simulink model "MIEM_Adaptive"  (Simulink 7.8)
settings: Solver=ode1  StartTime=0.0  StopTime=inf  FixedStep=0.001  RelTol=1e-3
undefined symbols (not defined in the file): HIL, qc_get_step_size
libraries: quarc_library x39, simulink x20, dspmtrx3 x3
(part 1 of 2)
settings Model: Creator=danso  LastModifiedBy=danso  SimulationMode=external  ExtModeTrigDuration=5000
settings SolverCC: PositivePriorityOrder=on
settings RTWCC: SystemTargetFile=quarc_win64.tlc  TemplateMakefile=quarc_default_tmf  Description=QUARC Win64 Target  ProcessScript=quarc_win64_make_rtw_hook
settings STFCustomTargetCC: TargetPreCompLibLocation=C:\PROGRA~3\QUARC\lib\2011b\win64\release  SystemTargetFile=quarc_win64.tlc
settings GRTTargetCC: TargetPreCompLibLocation=C:\PROGRA~3\QUARC\lib\2011b\win64\release  ParMdlRefBuildCompliant=off  CompOptLevelCompliant=off  ConcurrentExecutionCompliant=off  MatFileLogging=off  ExtMode=on  ExtModeMexFile=quarc_comm

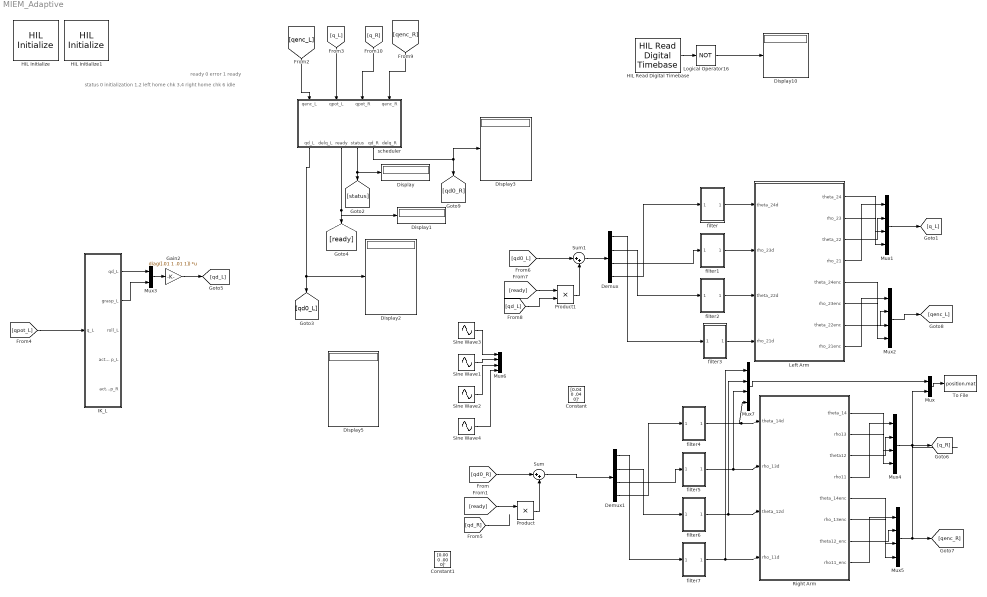
== system MIEM_Adaptive ==
  note: status
      | 0 initialization
      | 1,2 left home chk
      | 3,4 right home chk
      | 6 idle
  note: ready
      | 0 error
      | 1 ready
  Constant : Constant  Value=[0.04 0 .04 0]'
  Constant1 : Constant  Value=[0.00 0 .00 0]'
  Demux : Demux
  Demux1 : Demux
  Display{,1..3,5,10} (6 alike) : Display
  Gain2 : Gain  Gain=diag([.01 1 .01 1])  Multiplication=Matrix(K*u)
  HIL Initialize : quarc_library/Data Acquisition/Generic/Configuration/HIL Initialize  Priority=-99  object_name=HIL-1  board_type=qpid_e  board_number=0  board_options=enc0_dir=0;enc0_filter=1;enc0_a=1;enc0_b=1;enc0_z=0;enc0_reload=0;enc1_dir=0;enc1_filter=1;enc1_a=1;enc1_b=1;enc1_z=0;enc1_reload=0;enc2_dir=0;enc2_filter=1;enc2_a=1;enc2_b=1;enc2_z=0;enc2_reload=0;enc3_dir=0;enc3_filter=1;enc3_a=1;enc3_b=1;enc3_z=0;enc3_reload=0;enc4_dir=0;enc4_filter=1;enc4_a=1;enc4_b=1;enc4_z=0;enc4_reload=0;enc5_dir=0;enc5_filter=1;enc5_a=1;enc5_b=1;enc5_z=0;enc5_reload=0;enc6_dir=0;enc6_filter=1;enc6_a=1;enc6_b=1;enc6_z=0;enc6_reload=0;enc7_dir=0;enc7_filter=1;enc7_a=1;enc7_b=1;enc7_z=0;enc7_reload=0;ext_int_polarity=0;fuse_polarity=0;convert_polarity=0;watchdog_polarity=0;ext_int_watchdog=0;fuse_watchdog=0;trig1_watchdog=0;watchdog_to_trig1=0;watchdog_to_trig2=0;counter_to_trig0=0;trigger_adcs=0;latch_on_adc=0;pwm_immediate=0  exclusive=off  active=off  hardware_clocks=[0:16]  clock_modes=[]  initial_clock_frequencies=[]  set_clock_params_at_start=off  set_clock_params_at_switch_in=off  set_clock_frequencies_at_start=off  set_clock_frequencies_at_switch_in=off  analog_input_channels=[0:7]  analog_input_maximums=10  analog_input_minimums=-10  set_analog_input_params_at_start=off  set_analog_input_params_at_switch_in=off  analog_output_channels=[0:7]  analog_output_maximums=10  analog_output_minimums=-10  initial_analog_outputs=[0]  final_analog_outputs=[0]  watchdog_analog_outputs=0  set_analog_output_params_at_start=off  set_analog_output_params_at_switch_in=off  set_analog_outputs_at_start=on  set_analog_outputs_at_switch_in=off  set_analog_outputs_at_terminate=on  set_analog_outputs_at_switch_out=off  set_analog_outputs_on_watchdog=off  digital_input_channels=[]  digital_output_channels=[0:31 46:47 40:45 55]  digital_output_configuration=[]  initial_digital_outputs=[1]  final_digital_outputs=[1]  watchdog_digital_outputs=[2]  set_digital_output_params_at_start=off  set_digital_output_params_at_switch_in=off  set_digital_outputs_at_start=on  set_digital_outputs_at_switch_in=off  set_digital_outputs_at_terminate=on  set_digital_outputs_at_switch_out=off  set_digital_outputs_on_watchdog=off  encoder_channels=[0:7]  quadrature=4  encoder_filter_frequency=40e6/1  initial_encoder_counts=[0]  set_encoder_params_at_start=on  set_encoder_params_at_switch_in=off  set_encoder_counts_at_start=on  set_encoder_counts_at_switch_in=off  pwm_channels=[0:7]  pwm_modes=0  pwm_frequency=40e6/4096  pwm_configuration=[0]  pwm_alignment=[0]  pwm_polarity=[1]  pwm_leading_deadband=[0]  pwm_trailing_deadband=[0]  initial_pwm_outputs=[0]  final_pwm_outputs=[0]  watchdog_pwm_outputs=[0]  set_pwm_params_at_start=on  set_pwm_params_at_switch_in=off  set_pwm_outputs_at_start=on  set_pwm_outputs_at_switch_in=off  set_pwm_outputs_at_terminate=on  set_pwm_outputs_at_switch_out=off  set_pwm_outputs_on_watchdog=off  other_output_channels=[]  initial_other_outputs=[]  final_other_outputs=[]  watchdog_other_outputs=[]  set_other_outputs_at_start=off  set_other_outputs_at_switch_in=off  set_other_outputs_at_terminate=off  set_other_outputs_at_switch_out=off  set_other_outputs_on_watchdog=off
  HIL Initialize1 : quarc_library/Data Acquisition/Generic/Configuration/HIL Initialize  Priority=-99  object_name=HIL-2  board_type=qpid  board_number=0  board_options=enc0_dir=0;enc0_filter=1;enc0_a=1;enc0_b=1;enc0_z=0;enc0_reload=0;enc1_dir=0;enc1_filter=1;enc1_a=1;enc1_b=1;enc1_z=0;enc1_reload=0;enc2_dir=0;enc2_filter=1;enc2_a=1;enc2_b=1;enc2_z=0;enc2_reload=0;enc3_dir=0;enc3_filter=1;enc3_a=1;enc3_b=1;enc3_z=0;enc3_reload=0;enc4_dir=0;enc4_filter=1;enc4_a=1;enc4_b=1;enc4_z=0;enc4_reload=0;enc5_dir=0;enc5_filter=1;enc5_a=1;enc5_b=1;enc5_z=0;enc5_reload=0;enc6_dir=0;enc6_filter=1;enc6_a=1;enc6_b=1;enc6_z=0;enc6_reload=0;enc7_dir=0;enc7_filter=1;enc7_a=1;enc7_b=1;enc7_z=0;enc7_reload=0;ext_int_polarity=0;fuse_polarity=0;convert_polarity=0;watchdog_polarity=0;ext_int_watchdog=0;fuse_watchdog=0;trig1_watchdog=0;watchdog_to_trig1=0;watchdog_to_trig2=0;counter_to_trig0=0;trigger_adcs=0;latch_on_adc=0;pwm_immediate=0  exclusive=off  active=off  hardware_clocks=[0:16]  clock_modes=[]  initial_clock_frequencies=[]  set_clock_params_at_start=off  set_clock_params_at_switch_in=off  set_clock_frequencies_at_start=off  set_clock_frequencies_at_switch_in=off  analog_input_channels=[0:7]  analog_input_maximums=10  analog_input_minimums=-10  set_analog_input_params_at_start=off  set_analog_input_params_at_switch_in=off  analog_output_channels=[0:7]  analog_output_maximums=10  analog_output_minimums=-10  initial_analog_outputs=[0]  final_analog_outputs=[0]  watchdog_analog_outputs=0  set_analog_output_params_at_start=off  set_analog_output_params_at_switch_in=off  set_analog_outputs_at_start=on  set_analog_outputs_at_switch_in=off  set_analog_outputs_at_terminate=on  set_analog_outputs_at_switch_out=off  set_analog_outputs_on_watchdog=off  digital_input_channels=[48:55]  digital_output_channels=[]  digital_output_configuration=[]  initial_digital_outputs=[1]  final_digital_outputs=[1]  watchdog_digital_outputs=[2]  set_digital_output_params_at_start=off  set_digital_output_params_at_switch_in=off  set_digital_outputs_at_start=on  set_digital_outputs_at_switch_in=off  set_digital_outputs_at_terminate=on  set_digital_outputs_at_switch_out=off  set_digital_outputs_on_watchdog=off  encoder_channels=[0:7]  quadrature=[4]  encoder_filter_frequency=40e6/1  initial_encoder_counts=[0]  set_encoder_params_at_start=on  set_encoder_params_at_switch_in=off  set_encoder_counts_at_start=on  set_encoder_counts_at_switch_in=off  pwm_channels=[0:7]  pwm_modes=0  pwm_frequency=40e6/4096  pwm_configuration=[0]  pwm_alignment=[0]  pwm_polarity=[1]  pwm_leading_deadband=[0]  pwm_trailing_deadband=[0]  initial_pwm_outputs=[0]  final_pwm_outputs=[0]  watchdog_pwm_outputs=[0]  set_pwm_params_at_start=on  set_pwm_params_at_switch_in=off  set_pwm_outputs_at_start=on  set_pwm_outputs_at_switch_in=off  set_pwm_outputs_at_terminate=on  set_pwm_outputs_at_switch_out=off  set_pwm_outputs_on_watchdog=off  other_output_channels=[]  initial_other_outputs=[]  final_other_outputs=[]  watchdog_other_outputs=[]  set_other_outputs_at_start=off  set_other_outputs_at_switch_in=off  set_other_outputs_at_terminate=off  set_other_outputs_at_switch_out=off  set_other_outputs_on_watchdog=off
  HIL Read Digital Timebase : quarc_library/Data Acquisition/Generic/Timebases/HIL Read Digital Timebase  object_name=HIL-2  clock=0  channels=[48]  samples_in_buffer=max(ceil(1/qc_get_step_size), 1)  active=on  vector_output=off  data_type_mode=Inherit via back propagation  data_type=boolean
      settings: AttributesFormatString=(%<object_name>)
  IK_L : Subsystem
  Left Arm : Subsystem
  Logical Operator16 : Logic  Operator=NOT  AllPortsSameDT=off  OutDataTypeStr=boolean
  Mux : Mux  Inputs=2
  Mux{1..2,4..7} (6 alike) : Mux
  Mux3 : Mux  Inputs=[3 1]
  Product : Product  RndMeth=Zero
  Product1 : Product  RndMeth=Zero
  Right Arm : Subsystem
  Sine Wave1 : Sin  Amplitude=0  Frequency=.5  SampleTime=0
  Sine Wave2 : Sin  Amplitude=.0  Bias=.04  Frequency=.5  SampleTime=0
  Sine Wave3 : Sin  Amplitude=0  Bias=.04  Frequency=.5  SampleTime=0
  Sine Wave4 : Sin  Amplitude=0  Frequency=.5  SampleTime=0
  Sum : Sum  Inputs=|++
  Sum1 : Sum  Inputs=|++
  To File : ToFile  Filename=position.mat  MatrixName=x
  filter : Subsystem
  filter1 : Subsystem
  filter2 : Subsystem
  filter3 : Subsystem
  filter4 : Subsystem
  filter5 : Subsystem
  filter6 : Subsystem
  filter7 : Subsystem
  scheduler : Subsystem
  wires:
  Demux/3 -> filter1/1(In1)
  Demux/4 -> filter/1(In1)
  Demux/2 -> filter2/1(In1)
  filter3/1(Out1) -> Left Arm/4(rho_21d)
  filter2/1(Out1) -> Left Arm/3(theta_22d)
  filter1/1(Out1) -> Left Arm/2(rho_23d)
  filter/1(Out1) -> Left Arm/1(theta_24d)
  Demux/1 -> filter3/1(In1)
  scheduler/1(qd_L) -> [qd0_L], Display2/1
  [q_L] -> scheduler/2(qpot_L)
  [qenc_L] -> scheduler/1(qenc_L)
  [qd0_R] -> Sum/1
  Product/1 -> Sum/2
  [ready] -> Product/1
  IK_L/1(qd_L) -> Mux3/1
  IK_L/2(grasp_L) -> Mux3/2
  Mux3/1 -> Gain2/1
  Gain2/1 -> [qd_L]
  [qpot_L] -> IK_L/1(q_L)
  HIL Read Digital Timebase/1 -> Logical Operator16/1
  Logical Operator16/1 -> Display10/1
  filter4/1(Out1) -> Right Arm/1(theta_14d), Mux7/4
  filter5/1(Out1) -> Right Arm/2(rho_13d), Mux7/3
  filter6/1(Out1) -> Right Arm/3(theta_12d), Mux7/2
  filter7/1(Out1) -> Right Arm/4(rho_11d), Mux7/1
  Mux5/1 -> [qenc_R], Mux/2
  Mux4/1 -> [q_R]
  Right Arm/4(rho11) -> Mux4/1
  Right Arm/3(theta12) -> Mux4/2
  Right Arm/2(rho13) -> Mux4/3
  Right Arm/1(theta_14) -> Mux4/4
  Right Arm/8(rho11_enc) -> Mux5/1
  Right Arm/7(theta12_enc) -> Mux5/2
  Right Arm/6(rho_13enc) -> Mux5/3
  Right Arm/5(theta_14enc) -> Mux5/4
  Left Arm/4(rho_21) -> Mux1/1
  Left Arm/3(theta_22) -> Mux1/2
  Left Arm/2(rho_23) -> Mux1/3
  Left Arm/1(theta_24) -> Mux1/4
  Left Arm/8(rho_21enc) -> Mux2/1
  Left Arm/7(theta_22enc) -> Mux2/2
  Left Arm/6(rho_23enc) -> Mux2/3
  Left Arm/5(theta_24enc) -> Mux2/4
  Demux1/3 -> filter5/1(In1)
  Demux1/4 -> filter4/1(In1)
  Demux1/2 -> filter6/1(In1)
  Demux1/1 -> filter7/1(In1)
  Sum/1 -> Demux1/1
  [qd_R] -> ?
  Mux1/1 -> [q_L]
  Mux2/1 -> [qenc_L]
  [qd0_L] -> Sum1/1
  Product1/1 -> Sum1/2
  [ready] -> Product1/1
  Sum1/1 -> Demux/1
  scheduler/3(ready) -> [ready], Display1/1
  scheduler/4(status) -> [status], Display/1
  scheduler/5(qd_R) -> [qd0_R], Display3/1
  [q_R] -> scheduler/3(qpot_R)
  [qenc_R] -> scheduler/4(qenc_R)
  Mux/1 -> To File/1
  Sine Wave3/1 -> Mux6/1
  Sine Wave1/1 -> Mux6/2
  Sine Wave2/1 -> Mux6/3
  Sine Wave4/1 -> Mux6/4
  Mux7/1 -> Mux/1
  [qd_L] -> Product1/2

== system MIEM_Adaptive/IK_L ==
  q_L : Inport
  Derivative1 : Derivative
  Display : Display
  IK_L : Subsystem
  Memory : Memory
  Scope1 : Scope
      settings: YMin=-1.5  YMax=4  SaveName=ScopeData5
  filter : Subsystem
  phantom : Subsystem
  qd_L : Outport
  grasp_L : Outport  Port=2
  roll_L : Outport  Port=3
  actual p_L : Outport  Port=4
  actual p_R : Outport  Port=5
  wires:
  phantom/1(p) -> filter/1(In1)
  [F_left] -> Memory/1
  phantom/2(roll) -> roll_L/1
  phantom/3(grasp) -> grasp_L/1, Display/1
  [p_left] -> IK_L/1(In1), Derivative1/1
  Derivative1/1 -> IK_L/2(In2)
  IK_L/1(qd) -> qd_L/1
  IK_L/4(F) -> [F_left]
  Memory/1 -> phantom/1(boundary force)
  filter/1(Out1) -> [p_left]

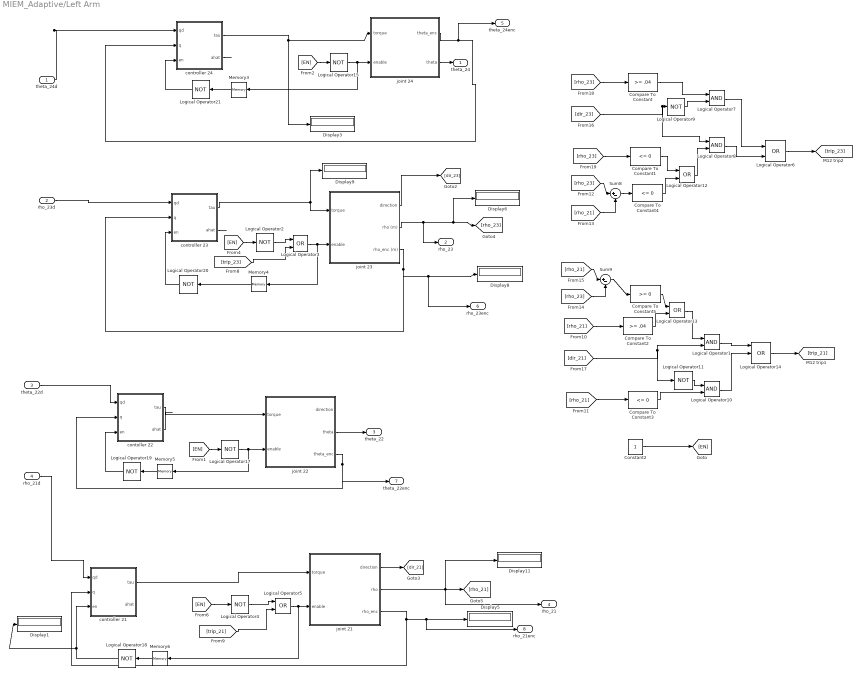
== system MIEM_Adaptive/Left Arm ==
  theta_24d : Inport
  rho_23d : Inport  Port=2
  theta_22d : Inport  Port=3
  rho_21d : Inport  Port=4
  Compare To Constant : simulink/Logic and Bit Operations/Compare To Constant  relop=>=  const=.04  OutDataTypeStr=uint8
  Compare To Constant1 : simulink/Logic and Bit Operations/Compare To Constant  relop=<=  const=0  OutDataTypeStr=uint8
  Compare To Constant2 : simulink/Logic and Bit Operations/Compare To Constant  relop=>=  const=.04  OutDataTypeStr=uint8
  Compare To Constant3 : simulink/Logic and Bit Operations/Compare To Constant  relop=<=  const=0  OutDataTypeStr=uint8
  Compare To Constant4 : simulink/Logic and Bit Operations/Compare To Constant  relop=<=  const=0  OutDataTypeStr=uint8
  Compare To Constant5 : simulink/Logic and Bit Operations/Compare To Constant  relop=>=  const=0  OutDataTypeStr=uint8
  Constant2 : Constant
  Display{1,3,5..6,8..9,11} (7 alike) : Display
  Logical Operator{1,7..8,10} (4 alike) : Logic  AllPortsSameDT=off  OutDataTypeStr=boolean
  Logical Operator{2,4,9,11,15,17..21} (10 alike) : Logic  Operator=NOT  AllPortsSameDT=off  OutDataTypeStr=boolean
  Logical Operator{3,5..6,12..13} (5 alike) : Logic  Operator=OR  AllPortsSameDT=off  OutDataTypeStr=boolean
  Logical Operator14 : Logic  Operator=OR  Inputs=3  AllPortsSameDT=off  OutDataTypeStr=boolean
  Memory{3..6} (4 alike) : Memory
  Sum8 : Sum  Inputs=|+-
  Sum9 : Sum  Inputs=|+-
  contoller 22 : Subsystem
  controller 21 : Subsystem
  controller 23 : Subsystem
  controller 24 : Subsystem
  joint 21 : Subsystem
  joint 22 : Subsystem
  joint 23 : Subsystem
  joint 24 : Subsystem
  theta_24 : Outport
  rho_23 : Outport  Port=2
  theta_22 : Outport  Port=3
  rho_21 : Outport  Port=4
  theta_24enc : Outport  Port=5
  rho_23enc : Outport  Port=6
  theta_22enc : Outport  Port=7
  rho_21enc : Outport  Port=8
  wires:
  Memory6/1 -> Logical Operator18/1
  Memory5/1 -> Logical Operator19/1
  [EN] -> Logical Operator4/1
  Logical Operator4/1 -> Logical Operator5/1
  [trip_21] -> Logical Operator5/2
  joint 21/2(rho) -> [rho_21], Display11/1, rho_21/1
  joint 22/3(theta_enc) -> theta_22enc/1, contoller 22/2(q)
  contoller 22/1(tau) -> joint 22/1(torque)
  Logical Operator17/1 -> joint 22/2(enable), Memory5/1
  [EN] -> Logical Operator17/1
  joint 21/1(direction) -> [dir_21]
  Logical Operator5/1 -> joint 21/2(enable), Memory6/1
  joint 21/3(rho_enc) -> Display5/1, rho_21enc/1, controller 21/2(q)
  joint 24/1(theta_enc) -> controller 24/2(q), theta_24enc/1
  controller 24/1(tau) -> Display3/1, joint 24/1(torque)
  [EN] -> Logical Operator2/1
  [trip_23] -> Logical Operator3/2
  Logical Operator2/1 -> Logical Operator3/1
  joint 23/1(direction) -> [dir_23]
  Logical Operator3/1 -> joint 23/2(enable), Memory4/1
  theta_24d/1 -> controller 24/1(qd)
  joint 23/2(rho (m)) -> [rho_23], Display6/1, rho_23/1
  joint 23/3(rho_enc (m)) -> controller 23/2(q), Display8/1, rho_23enc/1
  controller 23/1(tau) -> Display9/1, joint 23/1(torque)
  [EN] -> Logical Operator15/1
  Logical Operator15/1 -> joint 24/2(enable), Memory3/1
  Memory3/1 -> Logical Operator21/1
  Memory4/1 -> Logical Operator20/1
  controller 24/2(ahat) -> ?
  joint 24/2(theta) -> theta_24/1
  rho_23d/1 -> controller 23/1(qd)
  controller 23/2(ahat) -> ?
  theta_22d/1 -> contoller 22/1(qd)
  contoller 22/2(ahat) -> ?
  joint 22/2(theta) -> theta_22/1
  rho_21d/1 -> controller 21/1(qd)
  Logical Operator6/1 -> [trip_23]
  [dir_23] -> Logical Operator8/1, Logical Operator9/1
  Compare To Constant/1 -> Logical Operator7/1
  [rho_23] -> Compare To Constant1/1
  Logical Operator7/1 -> Logical Operator6/1
  Logical Operator8/1 -> Logical Operator6/2
  Logical Operator9/1 -> Logical Operator7/2
  [rho_23] -> Sum8/1
  [rho_21] -> Sum8/2
  Sum8/1 -> Compare To Constant4/1
  Compare To Constant4/1 -> Logical Operator12/2
  Compare To Constant1/1 -> Logical Operator12/1
  Logical Operator12/1 -> Logical Operator8/2
  [dir_21] -> Logical Operator11/1, Logical Operator1/2
  Compare To Constant3/1 -> Logical Operator10/2
  Logical Operator11/1 -> Logical Operator10/1
  [rho_21] -> Compare To Constant2/1
  [rho_21] -> Compare To Constant3/1
  Logical Operator13/1 -> Logical Operator1/1
  Compare To Constant2/1 -> Logical Operator13/2
  Sum9/1 -> Compare To Constant5/1
  [rho_21] -> Sum9/1
  [rho_23] -> Sum9/2
  Compare To Constant5/1 -> Logical Operator13/1
  Logical Operator1/1 -> Logical Operator14/1
  Logical Operator10/1 -> Logical Operator14/2
  Logical Operator14/1 -> [trip_21]
  Constant2/1 -> [EN]
  controller 21/1(tau) -> joint 21/1(torque)
  Logical Operator18/1 -> controller 21/3(en), Display1/1
  Logical Operator19/1 -> contoller 22/3(en)
  Logical Operator20/1 -> controller 23/3(en)
  Logical Operator21/1 -> controller 24/3(en)
  [rho_23] -> Compare To Constant/1

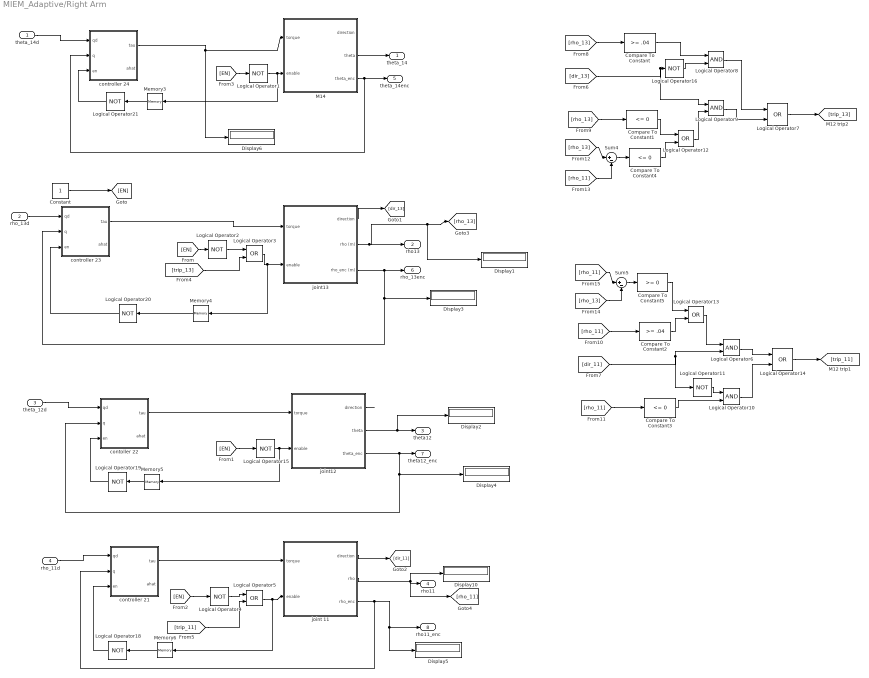
== system MIEM_Adaptive/Right Arm ==
  theta_14d : Inport
  rho_13d : Inport  Port=2
  theta_12d : Inport  Port=3
  rho_11d : Inport  Port=4
  Compare To Constant : simulink/Logic and Bit Operations/Compare To Constant  relop=>=  const=.04  OutDataTypeStr=uint8
  Compare To Constant1 : simulink/Logic and Bit Operations/Compare To Constant  relop=<=  const=0  OutDataTypeStr=uint8
  Compare To Constant2 : simulink/Logic and Bit Operations/Compare To Constant  relop=>=  const=.04  OutDataTypeStr=uint8
  Compare To Constant3 : simulink/Logic and Bit Operations/Compare To Constant  relop=<=  const=0  OutDataTypeStr=uint8
  Compare To Constant4 : simulink/Logic and Bit Operations/Compare To Constant  relop=<=  const=0  OutDataTypeStr=uint8
  Compare To Constant5 : simulink/Logic and Bit Operations/Compare To Constant  relop=>=  const=0  OutDataTypeStr=uint8
  Constant : Constant
  Display{1..6,10} (7 alike) : Display
  Logical Operator{1..2,4,11,15..16,18..21} (10 alike) : Logic  Operator=NOT  AllPortsSameDT=off  OutDataTypeStr=boolean
  Logical Operator{6,8..10} (4 alike) : Logic  AllPortsSameDT=off  OutDataTypeStr=boolean
  Logical Operator{3,5,7,12..14} (6 alike) : Logic  Operator=OR  AllPortsSameDT=off  OutDataTypeStr=boolean
  M14 : Subsystem
  Memory{3..6} (4 alike) : Memory
  Sum4 : Sum  Inputs=|+-
  Sum5 : Sum  Inputs=|+-
  contoller 22 : Subsystem
  controller 21 : Subsystem
  controller 23 : Subsystem
  controller 24 : Subsystem
  joint 11 : Subsystem
  joint12 : Subsystem
  joint13 : Subsystem
  theta_14 : Outport
  rho13 : Outport  Port=2
  theta12 : Outport  Port=3
  rho11 : Outport  Port=4
  theta_14enc : Outport  Port=5
  rho_13enc : Outport  Port=6
  theta12_enc : Outport  Port=7
  rho11_enc : Outport  Port=8
  wires:
  Constant/1 -> [EN]
  [EN] -> Logical Operator2/1
  Logical Operator3/1 -> joint13/2(enable), Memory4/1
  [trip_13] -> Logical Operator3/2
  Logical Operator2/1 -> Logical Operator3/1
  joint13/1(direction) -> [dir_13]
  controller 23/1(tau) -> joint13/1(torque)
  joint13/2(rho (m)) -> rho13/1, [rho_13], Display1/1
  joint13/3(rho_enc (m)) -> Display3/1, controller 23/2(q), rho_13enc/1
  Memory4/1 -> Logical Operator20/1
  Logical Operator20/1 -> controller 23/3(en)
  [EN] -> Logical Operator15/1
  Logical Operator15/1 -> joint12/2(enable), Memory5/1
  joint12/3(theta_enc) -> Display4/1, contoller 22/2(q), theta12_enc/1
  joint12/2(theta) -> theta12/1, Display2/1
  Memory5/1 -> Logical Operator19/1
  Logical Operator19/1 -> contoller 22/3(en)
  contoller 22/1(tau) -> joint12/1(torque)
  [trip_11] -> Logical Operator5/2
  Logical Operator4/1 -> Logical Operator5/1
  [EN] -> Logical Operator4/1
  Logical Operator5/1 -> joint 11/2(enable), Memory6/1
  joint 11/1(direction) -> [dir_11]
  joint 11/3(rho_enc) -> Display5/1, rho11_enc/1, controller 21/2(q)
  joint 11/2(rho) -> rho11/1, Display10/1, [rho_11]
  controller 21/1(tau) -> joint 11/1(torque)
  Memory6/1 -> Logical Operator18/1
  Logical Operator18/1 -> controller 21/3(en)
  M14/2(theta) -> theta_14/1
  controller 24/1(tau) -> Display6/1, M14/1(torque)
  [EN] -> Logical Operator1/1
  Logical Operator1/1 -> Memory3/1, M14/2(enable)
  Memory3/1 -> Logical Operator21/1
  M14/3(theta_enc) -> controller 24/2(q), theta_14enc/1
  Logical Operator21/1 -> controller 24/3(en)
  theta_14d/1 -> controller 24/1(qd)
  rho_13d/1 -> controller 23/1(qd)
  theta_12d/1 -> contoller 22/1(qd)
  rho_11d/1 -> controller 21/1(qd)
  joint12/1(direction) -> ?
  Logical Operator7/1 -> [trip_13]
  [dir_13] -> Logical Operator9/1, Logical Operator16/1
  Compare To Constant/1 -> Logical Operator8/1
  [rho_13] -> Compare To Constant/1
  [rho_13] -> Compare To Constant1/1
  [dir_11] -> Logical Operator11/1, Logical Operator6/2
  Compare To Constant3/1 -> Logical Operator10/2
  Logical Operator11/1 -> Logical Operator10/1
  [rho_11] -> Compare To Constant2/1
  [rho_11] -> Compare To Constant3/1
  Logical Operator8/1 -> Logical Operator7/1
  Logical Operator9/1 -> Logical Operator7/2
  Logical Operator16/1 -> Logical Operator8/2
  [rho_13] -> Sum4/1
  [rho_11] -> Sum4/2
  Sum4/1 -> Compare To Constant4/1
  Compare To Constant4/1 -> Logical Operator12/2
  Compare To Constant1/1 -> Logical Operator12/1
  Logical Operator12/1 -> Logical Operator9/2
  Logical Operator13/1 -> Logical Operator6/1
  Compare To Constant2/1 -> Logical Operator13/2
  Sum5/1 -> Compare To Constant5/1
  [rho_11] -> Sum5/1
  [rho_13] -> Sum5/2
  Compare To Constant5/1 -> Logical Operator13/1
  Logical Operator6/1 -> Logical Operator14/1
  Logical Operator10/1 -> Logical Operator14/2
  Logical Operator14/1 -> [trip_11]

== system MIEM_Adaptive/filter ==
  In1 : Inport
  Memory : Memory
  filter : MATLAB Function  TreatAsAtomicUnit=on
  Out1 : Outport
  wires:
  filter/1(y) -> Memory/1, Out1/1
  Memory/1 -> filter/2(u_)
  In1/1 -> filter/1(u)

== system MIEM_Adaptive/filter1 ==
  In1 : Inport
  Memory : Memory
  filter : MATLAB Function  TreatAsAtomicUnit=on
  Out1 : Outport
  wires:
  filter/1(y) -> Memory/1, Out1/1
  Memory/1 -> filter/2(u_)
  In1/1 -> filter/1(u)

== system MIEM_Adaptive/filter2 ==
  In1 : Inport
  Memory : Memory
  filter : MATLAB Function  TreatAsAtomicUnit=on
  Out1 : Outport
  wires:
  filter/1(y) -> Memory/1, Out1/1
  Memory/1 -> filter/2(u_)
  In1/1 -> filter/1(u)

== system MIEM_Adaptive/filter3 ==
  In1 : Inport
  Memory : Memory
  filter : MATLAB Function  TreatAsAtomicUnit=on
  Out1 : Outport
  wires:
  filter/1(y) -> Memory/1, Out1/1
  Memory/1 -> filter/2(u_)
  In1/1 -> filter/1(u)

== system MIEM_Adaptive/filter4 ==
  In1 : Inport
  Memory : Memory
  filter : MATLAB Function  TreatAsAtomicUnit=on
  Out1 : Outport
  wires:
  filter/1(y) -> Memory/1, Out1/1
  Memory/1 -> filter/2(u_)
  In1/1 -> filter/1(u)

== system MIEM_Adaptive/filter5 ==
  In1 : Inport
  Memory : Memory
  filter : MATLAB Function  TreatAsAtomicUnit=on
  Out1 : Outport
  wires:
  filter/1(y) -> Memory/1, Out1/1
  Memory/1 -> filter/2(u_)
  In1/1 -> filter/1(u)

== system MIEM_Adaptive/filter6 ==
  In1 : Inport
  Memory : Memory
  filter : MATLAB Function  TreatAsAtomicUnit=on
  Out1 : Outport
  wires:
  filter/1(y) -> Memory/1, Out1/1
  Memory/1 -> filter/2(u_)
  In1/1 -> filter/1(u)

== system MIEM_Adaptive/filter7 ==
  In1 : Inport
  Memory : Memory
  filter : MATLAB Function  TreatAsAtomicUnit=on
  Out1 : Outport
  wires:
  filter/1(y) -> Memory/1, Out1/1
  Memory/1 -> filter/2(u_)
  In1/1 -> filter/1(u)

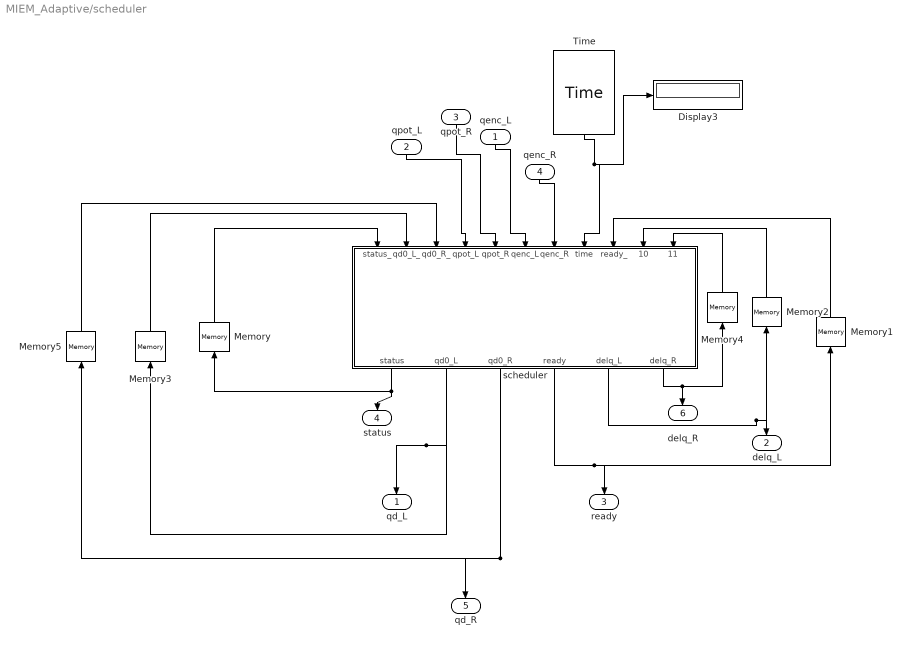
== system MIEM_Adaptive/scheduler ==
  qenc_L : Inport
  qpot_L : Inport  Port=2
  qpot_R : Inport  Port=3
  qenc_R : Inport  Port=4
  Display3 : Display
  Memory : Memory
  Memory1 : Memory
  Memory{2..5} (4 alike) : Memory  X0=[0 0 0 0]'
  Time : quarc_library/Sources/Time/Time  sample_time=qc_get_step_size
  scheduler : MATLAB Function  TreatAsAtomicUnit=on
  qd_L : Outport
  delq_L : Outport  Port=2
  ready : Outport  Port=3
  status : Outport  Port=4
  qd_R : Outport  Port=5
  delq_R : Outport  Port=6
  wires:
  Time/1 -> scheduler/8(time), Display3/1
  scheduler/1(status) -> Memory/1, status/1
  Memory/1 -> scheduler/1(status_)
  scheduler/4(ready) -> Memory1/1, ready/1
  Memory1/1 -> scheduler/9(ready_)
  qenc_L/1 -> scheduler/6(qenc_L)
  qpot_L/1 -> scheduler/4(qpot_L)
  scheduler/2(qd0_L) -> qd_L/1, Memory3/1
  Memory2/1 -> scheduler/10(delq_L_)
  scheduler/5(delq_L) -> Memory2/1, delq_L/1
  Memory3/1 -> scheduler/2(qd0_L_)
  scheduler/6(delq_R) -> Memory4/1, delq_R/1
  Memory4/1 -> scheduler/11(delq_R_)
  Memory5/1 -> scheduler/3(qd0_R_)
  scheduler/3(qd0_R) -> Memory5/1, qd_R/1
  qpot_R/1 -> scheduler/5(qpot_R)
  qenc_R/1 -> scheduler/7(qenc_R)

== system MIEM_Adaptive/IK_L/IK_L ==
  In1 : Inport
  In2 : Inport  Port=2
  Gain5 : Gain  Gain=[0 0 -1;-1 0 0;0 1 0]  Multiplication=Matrix(K*u)
  IK : MATLAB Function  TreatAsAtomicUnit=on
  Integrator : Integrator
  Memory1 : Memory  X0=[0 0 0]'
  Memory3 : Memory
  Memory4 : Memory
  qd : Outport
  Out2 : Outport  Port=2
  Out3 : Outport  Port=3
  F : Outport  Port=4
  wires:
  Memory1/1 -> IK/1(q_)
  IK/1(q) -> Memory1/1
  IK/5(F) -> Gain5/1
  IK/6(k) -> Memory3/1
  Memory3/1 -> IK/4(k_)
  IK/3(qdot) -> Integrator/1
  IK/2(qm) -> qd/1
  IK/7(r) -> Memory4/1
  Memory4/1 -> IK/5(r_)
  In1/1 -> IK/2(pd)
  Integrator/1 -> Out2/1
  In2/1 -> IK/3(pd_d)
  IK/4(error) -> Out3/1
  Gain5/1 -> F/1

== system MIEM_Adaptive/IK_L/filter ==
  In1 : Inport
  Demux : Demux  Outputs=3
  Mux : Mux  Inputs=3
  Transfer Fcn : TransferFcn  Denominator=[.2 1]
  Transfer Fcn1 : TransferFcn  Denominator=[.2 1]
  Transfer Fcn2 : TransferFcn  Denominator=[.2 1]
  Out1 : Outport
  wires:
  Transfer Fcn/1 -> Mux/1
  Transfer Fcn1/1 -> Mux/2
  Transfer Fcn2/1 -> Mux/3
  Demux/1 -> Transfer Fcn/1
  Demux/2 -> Transfer Fcn1/1
  Demux/3 -> Transfer Fcn2/1
  Mux/1 -> Out1/1
  In1/1 -> Demux/1

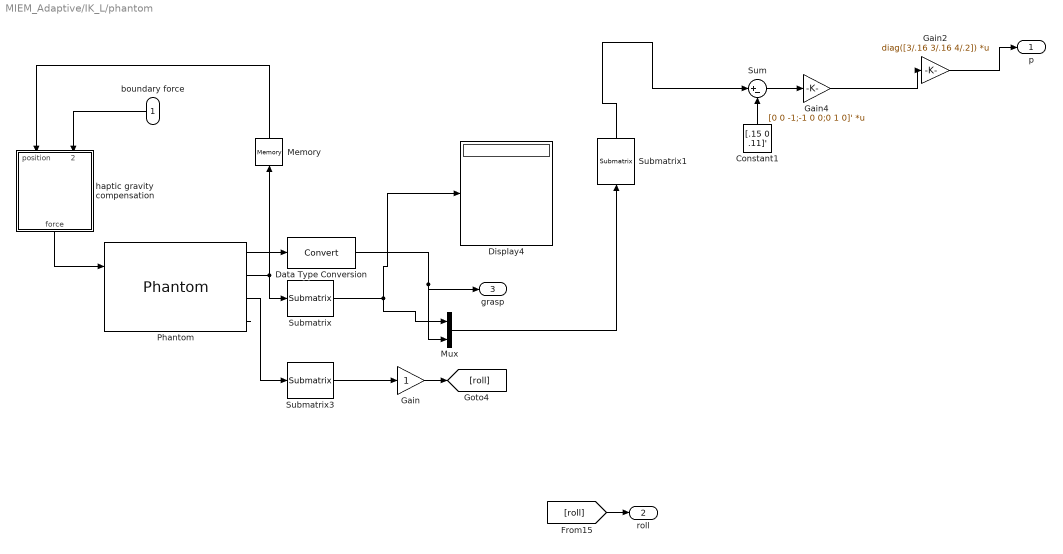
== system MIEM_Adaptive/IK_L/phantom ==
  boundary force : Inport
  Constant1 : Constant  Value=[.15 0 .11]'
  Data Type Conversion : DataTypeConversion
  Display4 : Display
  Gain : Gain
  Gain2 : Gain  Gain=diag([3/.16 3/.16 4/.2])  Multiplication=Matrix(K*u)
  Gain4 : Gain  Gain=[0 0 -1;-1 0 0;0 1 0]'  Multiplication=Matrix(K*u)
  Memory : Memory
  Mux : Mux  Inputs=2
  Phantom : quarc_library/Devices/Third-Party/SensAble/Phantom/Phantom  device_name=Default PHANToM  output_type=Positions and Gimbal Angles  input_type=Cartesian space  velocity_limit_option=on  velocity_limit=1200  is_7dof=off  sample_time=-1
      settings: AttributesFormatString=(%<device_name>)
  Submatrix : dspmtrx3/Submatrix  RowSpan=Range of rows  RowStartMode=First  RowStartIndex=1  RowEndMode=Index  RowEndIndex=3  ColSpan=Range of columns  ColStartMode=First  ColStartIndex=1  ColEndMode=Last  ColEndIndex=1
  Submatrix1 : dspmtrx3/Submatrix  RowSpan=Range of rows  RowStartMode=First  RowStartIndex=1  RowEndMode=Index  RowEndIndex=3  ColSpan=Range of columns  ColStartMode=First  ColStartIndex=1  ColEndMode=Last  ColEndIndex=1
  Submatrix3 : dspmtrx3/Submatrix  RowSpan=Range of rows  RowStartMode=Last  RowStartIndex=1  RowEndMode=Index  RowEndIndex=3  ColSpan=All columns  ColStartMode=First  ColStartIndex=1  ColEndMode=Last  ColEndIndex=1
  Sum : Sum  Inputs=|+-
  haptic gravity compensation : Subsystem
  p : Outport
  roll : Outport  Port=2
  grasp : Outport  Port=3
  wires:
  Phantom/2 -> Submatrix/1, Memory/1
  Submatrix/1 -> Display4/1, Mux/1
  Phantom/1 -> Data Type Conversion/1
  Data Type Conversion/1 -> Mux/2, grasp/1
  Submatrix1/1 -> Sum/1
  Mux/1 -> Submatrix1/1
  Submatrix3/1 -> Gain/1
  Phantom/3 -> Submatrix3/1
  Gain/1 -> [roll]
  Gain2/1 -> p/1
  Phantom/4 -> ?
  [roll] -> roll/1
  haptic gravity compensation/1(force) -> Phantom/1
  boundary force/1 -> haptic gravity compensation/2(boundary force)
  Memory/1 -> haptic gravity compensation/1(position)
  Constant1/1 -> Sum/2
  Sum/1 -> Gain4/1
  Gain4/1 -> Gain2/1

== system MIEM_Adaptive/Left Arm/contoller 22 ==
  qd : Inport
  q : Inport  Port=2
  en : Inport  Port=3
  Constant : Constant  Value=15
  Constant1 : Constant  Value=1e9
  Derivative3 : Derivative
  Derivative4 : Derivative
  Derivative5 : Derivative
  Memory3 : Memory  X0="[-0.0083    0.0320    0.0169   -0.2088]'"
  slotine's adaptive : MATLAB Function  TreatAsAtomicUnit=on
  tau : Outport
  ahat : Outport  Port=2
  wires:
  Derivative4/1 -> slotine's adaptive/6(qddotdot)
  Derivative5/1 -> slotine's adaptive/8(qdot)
  Derivative3/1 -> Derivative4/1, slotine's adaptive/5(qddot)
  slotine's adaptive/2(ahat) -> Memory3/1, ahat/1
  Memory3/1 -> slotine's adaptive/9(ahat_)
  Constant/1 -> slotine's adaptive/2(lambda)
  Constant1/1 -> slotine's adaptive/3(gamma)
  qd/1 -> slotine's adaptive/4(qd), Derivative3/1
  q/1 -> slotine's adaptive/7(q), Derivative5/1
  slotine's adaptive/1(tau) -> tau/1
  en/1 -> slotine's adaptive/1(en)

== system MIEM_Adaptive/Left Arm/controller 21 ==
  qd : Inport
  q : Inport  Port=2
  en : Inport  Port=3
  Constant : Constant  Value=100
  Constant1 : Constant  Value=1e10
  Derivative3 : Derivative
  Derivative4 : Derivative
  Derivative5 : Derivative
  Memory3 : Memory  X0="[2.4504    0.2033    0.3366    0.1727  -10.4533]'"
  slotine's adaptive : MATLAB Function  TreatAsAtomicUnit=on
  tau : Outport
  ahat : Outport  Port=2
  wires:
  Derivative4/1 -> slotine's adaptive/6(qddotdot)
  Derivative5/1 -> slotine's adaptive/8(qdot)
  Derivative3/1 -> Derivative4/1, slotine's adaptive/5(qddot)
  slotine's adaptive/2(ahat) -> Memory3/1, ahat/1
  Memory3/1 -> slotine's adaptive/9(ahat_)
  Constant/1 -> slotine's adaptive/2(lambda)
  Constant1/1 -> slotine's adaptive/3(gamma)
  qd/1 -> slotine's adaptive/4(qd), Derivative3/1
  q/1 -> slotine's adaptive/7(q), Derivative5/1
  slotine's adaptive/1(tau) -> tau/1
  en/1 -> slotine's adaptive/1(en)

== system MIEM_Adaptive/Left Arm/controller 23 ==
  qd : Inport
  q : Inport  Port=2
  en : Inport  Port=3
  Constant : Constant  Value=90
  Constant1 : Constant  Value=1e6
  Derivative3 : Derivative
  Derivative4 : Derivative
  Derivative5 : Derivative
  Memory3 : Memory  X0="[ 2.4073    0.0972    0.0790   -5.3481]'"
  slotine's adaptive : MATLAB Function  TreatAsAtomicUnit=on
  tau : Outport
  ahat : Outport  Port=2
  wires:
  Derivative4/1 -> slotine's adaptive/6(qddotdot)
  Derivative5/1 -> slotine's adaptive/8(qdot)
  Derivative3/1 -> Derivative4/1, slotine's adaptive/5(qddot)
  slotine's adaptive/2(ahat) -> Memory3/1, ahat/1
  Memory3/1 -> slotine's adaptive/9(ahat_)
  Constant/1 -> slotine's adaptive/2(lambda)
  Constant1/1 -> slotine's adaptive/3(gamma)
  qd/1 -> slotine's adaptive/4(qd), Derivative3/1
  q/1 -> slotine's adaptive/7(q), Derivative5/1
  slotine's adaptive/1(tau) -> tau/1
  en/1 -> slotine's adaptive/1(en)

== system MIEM_Adaptive/Left Arm/controller 24 ==
  qd : Inport
  q : Inport  Port=2
  en : Inport  Port=3
  Constant : Constant  Value=50
  Constant1 : Constant  Value=1e6
  Derivative3 : Derivative
  Derivative4 : Derivative
  Derivative5 : Derivative
  Memory3 : Memory  X0="[0.0008    0.0273    0.0390   -0.0832]'"
  slotine's adaptive : MATLAB Function  TreatAsAtomicUnit=on
  tau : Outport
  ahat : Outport  Port=2
  wires:
  Derivative4/1 -> slotine's adaptive/6(qddotdot)
  Derivative5/1 -> slotine's adaptive/8(qdot)
  Derivative3/1 -> Derivative4/1, slotine's adaptive/5(qddot)
  slotine's adaptive/2(ahat) -> Memory3/1, ahat/1
  Memory3/1 -> slotine's adaptive/9(ahat_)
  Constant/1 -> slotine's adaptive/2(lambda)
  Constant1/1 -> slotine's adaptive/3(gamma)
  qd/1 -> slotine's adaptive/4(qd), Derivative3/1
  q/1 -> slotine's adaptive/7(q), Derivative5/1
  slotine's adaptive/1(tau) -> tau/1
  en/1 -> slotine's adaptive/1(en)

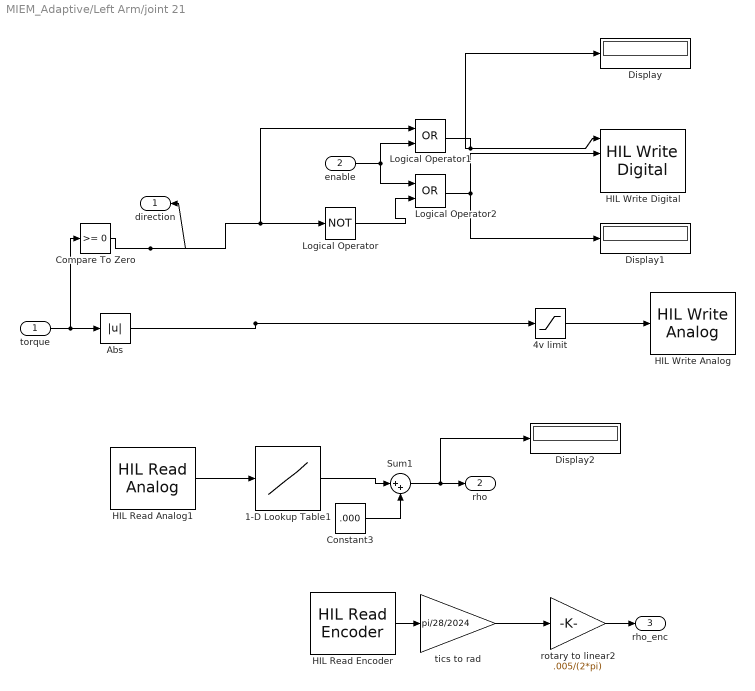
== system MIEM_Adaptive/Left Arm/joint 21 ==
  torque : Inport
  enable : Inport  Port=2
  1-D Lookup Table1 : Lookup_n-D  NumberOfTableDimensions=1  BreakpointsForDimension1=[.14 .26 .4 .66 .92 1.21 1.59 2.49 3.63]  Table=[0.0:.005:.04]  RndMeth=Simplest  InputSameDT=on
  4v limit : Saturate  UpperLimit=4  LowerLimit=0
  Abs : Abs
  Compare To Zero : simulink/Logic and Bit Operations/Compare To Zero  relop=>=  OutDataTypeStr=boolean
  Constant3 : Constant  Value=.000
  Display : Display
  Display1 : Display
  Display2 : Display
  HIL Read Analog1 : quarc_library/Data Acquisition/Generic/Immediate I//O/HIL Read Analog  object_name=HIL-2  channels=[7]  sample_time=qc_get_step_size  active=on  vector_output=off
  HIL Read Encoder : quarc_library/Data Acquisition/Generic/Immediate I//O/HIL Read Encoder  object_name=HIL-2  channels=[4]  sample_time=qc_get_step_size  active=on  vector_output=off  data_type_mode=Inherit via back propagation  data_type=double
  HIL Write Analog : quarc_library/Data Acquisition/Generic/Immediate I//O/HIL Write Analog  object_name=HIL-1  channels=[4]  sample_time=-1  active=off  vector_input=off
  HIL Write Digital : quarc_library/Data Acquisition/Generic/Immediate I//O/HIL Write Digital  object_name=HIL-1  channels=[16:19]  sample_time=-1  active=off  vector_input=off
  Logical Operator : Logic  Operator=NOT  AllPortsSameDT=off  OutDataTypeStr=boolean
  Logical Operator1 : Logic  Operator=OR  AllPortsSameDT=off  OutDataTypeStr=boolean
  Logical Operator2 : Logic  Operator=OR  AllPortsSameDT=off  OutDataTypeStr=boolean
  Sum1 : Sum  Inputs=|++
  rotary to linear2 : Gain  Gain=.005/(2*pi)
  tics to rad : Gain  Gain=pi/28/2024
  direction : Outport
  rho : Outport  Port=2
  rho_enc : Outport  Port=3
  wires:
  4v limit/1 -> HIL Write Analog/1
  Compare To Zero/1 -> direction/1, Logical Operator/1, Logical Operator1/1
  Abs/1 -> 4v limit/1
  torque/1 -> Abs/1, Compare To Zero/1
  HIL Read Analog1/1 -> 1-D Lookup Table1/1
  Logical Operator/1 -> Logical Operator2/2
  enable/1 -> Logical Operator1/2, Logical Operator2/1
  Logical Operator1/1 -> Display/1, HIL Write Digital/1
  Logical Operator2/1 -> Display1/1, HIL Write Digital/2
  tics to rad/1 -> rotary to linear2/1
  rotary to linear2/1 -> rho_enc/1
  HIL Read Encoder/1 -> tics to rad/1
  1-D Lookup Table1/1 -> Sum1/1
  Constant3/1 -> Sum1/2
  Sum1/1 -> rho/1, Display2/1

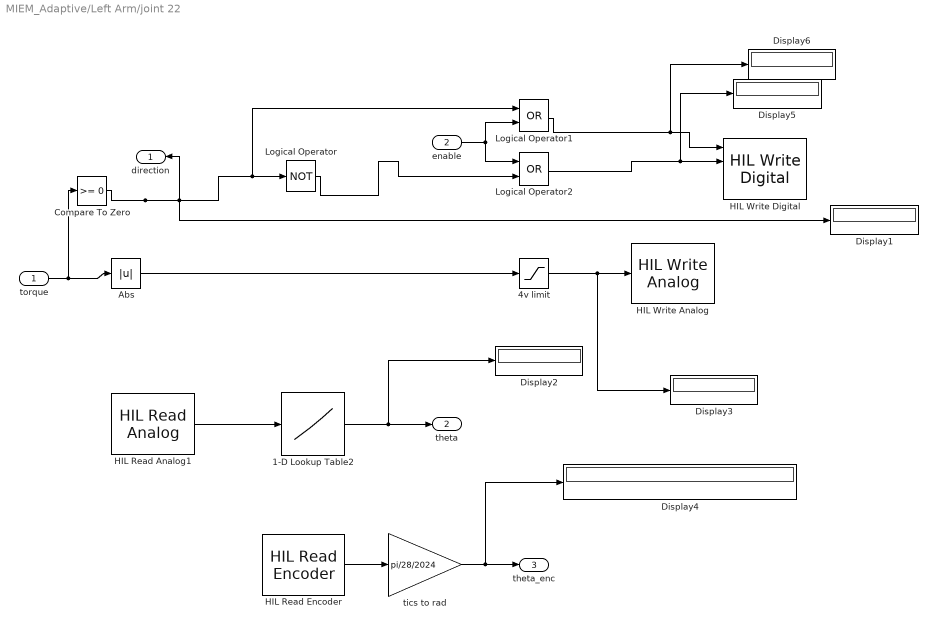
== system MIEM_Adaptive/Left Arm/joint 22 ==
  torque : Inport
  enable : Inport  Port=2
  1-D Lookup Table2 : Lookup_n-D  NumberOfTableDimensions=1  BreakpointsForDimension1=[.81 1.71 2.55 3.41 4.32]  Table=[2 1 0 -1 -2]  RndMeth=Simplest  InputSameDT=on
  4v limit : Saturate  UpperLimit=4  LowerLimit=0
  Abs : Abs
  Compare To Zero : simulink/Logic and Bit Operations/Compare To Zero  relop=>=  OutDataTypeStr=boolean
  Display{1..6} (6 alike) : Display
  HIL Read Analog1 : quarc_library/Data Acquisition/Generic/Immediate I//O/HIL Read Analog  object_name=HIL-1  channels=[5]  sample_time=qc_get_step_size  active=on  vector_output=off
  HIL Read Encoder : quarc_library/Data Acquisition/Generic/Immediate I//O/HIL Read Encoder  object_name=HIL-2  channels=[5]  sample_time=qc_get_step_size  active=on  vector_output=off  data_type_mode=Inherit via back propagation  data_type=double
  HIL Write Analog : quarc_library/Data Acquisition/Generic/Immediate I//O/HIL Write Analog  object_name=HIL-1  channels=[5]  sample_time=-1  active=off  vector_input=off
  HIL Write Digital : quarc_library/Data Acquisition/Generic/Immediate I//O/HIL Write Digital  object_name=HIL-1  channels=[20:23]  sample_time=-1  active=off  vector_input=off
  Logical Operator : Logic  Operator=NOT  AllPortsSameDT=off  OutDataTypeStr=boolean
  Logical Operator1 : Logic  Operator=OR  AllPortsSameDT=off  OutDataTypeStr=boolean
  Logical Operator2 : Logic  Operator=OR  AllPortsSameDT=off  OutDataTypeStr=boolean
  tics to rad : Gain  Gain=pi/28/2024
  direction : Outport
  theta : Outport  Port=2
  theta_enc : Outport  Port=3
  wires:
  4v limit/1 -> HIL Write Analog/1, Display3/1
  Compare To Zero/1 -> Logical Operator/1, Logical Operator1/1, direction/1, Display1/1
  Abs/1 -> 4v limit/1
  torque/1 -> Abs/1, Compare To Zero/1
  HIL Read Analog1/1 -> 1-D Lookup Table2/1
  HIL Read Encoder/1 -> tics to rad/1
  Logical Operator/1 -> Logical Operator2/2
  Logical Operator1/1 -> HIL Write Digital/1, Display6/1
  Logical Operator2/1 -> HIL Write Digital/2, Display5/1
  enable/1 -> Logical Operator1/2, Logical Operator2/1
  tics to rad/1 -> theta_enc/1, Display4/1
  1-D Lookup Table2/1 -> Display2/1, theta/1

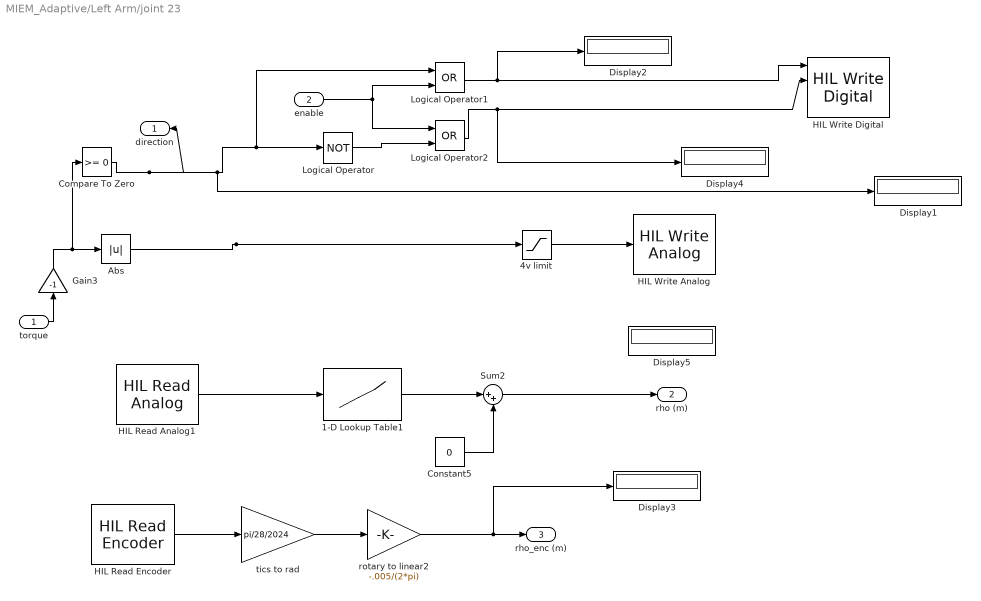
== system MIEM_Adaptive/Left Arm/joint 23 ==
  torque : Inport
  enable : Inport  Port=2
  1-D Lookup Table1 : Lookup_n-D  NumberOfTableDimensions=1  BreakpointsForDimension1=[.133 .1965 .272 .3497 .4297 .502 .587 .6821 .7468 .929 1.061 1.251 1.405 1.579 1.86 2.025 2.228 2.407 2.617 2.802 3.002 3.193 3.437 3.611 3.746 3.866]  Table=[.04 .0366 .0341 .032 .034 .029 .02746 .0256 .0243 .02016 .01821 .01519 .013 .01098 .0084 .00747 .0066 .00597 .00494 .004179 .00334 .00254 .00156 .00081 .00013 0]  RndMeth=Simplest  InputSameDT=on
  4v limit : Saturate  UpperLimit=4  LowerLimit=0
  Abs : Abs
  Compare To Zero : simulink/Logic and Bit Operations/Compare To Zero  relop=>=  OutDataTypeStr=boolean
  Constant5 : Constant  Value=0
  Display{1..5} (5 alike) : Display
  Gain3 : Gain  Gain=-1
  HIL Read Analog1 : quarc_library/Data Acquisition/Generic/Immediate I//O/HIL Read Analog  object_name=HIL-2  channels=[6]  sample_time=qc_get_step_size  active=on  vector_output=off
  HIL Read Encoder : quarc_library/Data Acquisition/Generic/Immediate I//O/HIL Read Encoder  object_name=HIL-2  channels=[6]  sample_time=qc_get_step_size  active=on  vector_output=off  data_type_mode=Inherit via back propagation  data_type=double
  HIL Write Analog : quarc_library/Data Acquisition/Generic/Immediate I//O/HIL Write Analog  object_name=HIL-1  channels=[6]  sample_time=-1  active=off  vector_input=off
  HIL Write Digital : quarc_library/Data Acquisition/Generic/Immediate I//O/HIL Write Digital  object_name=HIL-1  channels=[24:27]  sample_time=-1  active=off  vector_input=off
  Logical Operator : Logic  Operator=NOT  AllPortsSameDT=off  OutDataTypeStr=boolean
  Logical Operator1 : Logic  Operator=OR  AllPortsSameDT=off  OutDataTypeStr=boolean
  Logical Operator2 : Logic  Operator=OR  AllPortsSameDT=off  OutDataTypeStr=boolean
  Sum2 : Sum  Inputs=|++
  rotary to linear2 : Gain  Gain=-.005/(2*pi)
  tics to rad : Gain  Gain=pi/28/2024
  direction : Outport
  rho (m) : Outport  Port=2
  rho_enc (m) : Outport  Port=3
  wires:
  4v limit/1 -> HIL Write Analog/1
  Compare To Zero/1 -> direction/1, Logical Operator1/1, Logical Operator/1, Display1/1
  Abs/1 -> 4v limit/1
  torque/1 -> Gain3/1
  HIL Read Encoder/1 -> tics to rad/1
  ? -> ?
  Logical Operator1/1 -> Display2/1, HIL Write Digital/1
  Logical Operator2/1 -> Display4/1, HIL Write Digital/2
  enable/1 -> Logical Operator1/2, Logical Operator2/1
  tics to rad/1 -> rotary to linear2/1
  rotary to linear2/1 -> rho_enc (m)/1, Display3/1
  HIL Read Analog1/1 -> 1-D Lookup Table1/1
  1-D Lookup Table1/1 -> Sum2/1
  Constant5/1 -> Sum2/2
  Sum2/1 -> rho (m)/1
  Logical Operator/1 -> Logical Operator2/2
  Gain3/1 -> Abs/1, Compare To Zero/1

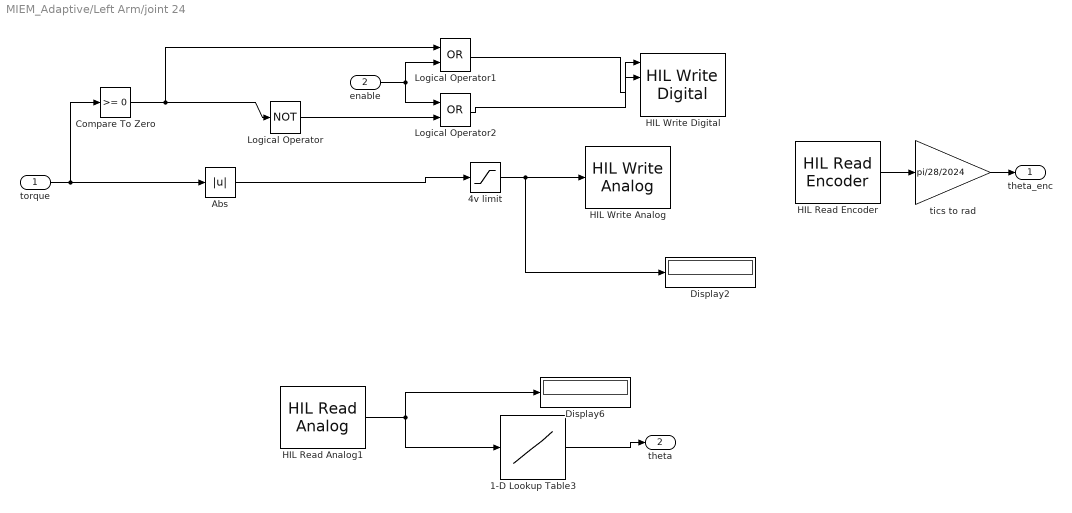
== system MIEM_Adaptive/Left Arm/joint 24 ==
  torque : Inport
  enable : Inport  Port=2
  1-D Lookup Table3 : Lookup_n-D  NumberOfTableDimensions=1  BreakpointsForDimension1=[.94 1.45 2.23 3.02 3.52]  Table=[pi/2 1 0 -1 -pi/2]  RndMeth=Simplest  InputSameDT=on
  4v limit : Saturate  UpperLimit=4  LowerLimit=0
  Abs : Abs
  Compare To Zero : simulink/Logic and Bit Operations/Compare To Zero  relop=>=  OutDataTypeStr=boolean
  Display2 : Display
  Display6 : Display
  HIL Read Analog1 : quarc_library/Data Acquisition/Generic/Immediate I//O/HIL Read Analog  object_name=HIL-1  channels=[7]  sample_time=qc_get_step_size  active=on  vector_output=off
  HIL Read Encoder : quarc_library/Data Acquisition/Generic/Immediate I//O/HIL Read Encoder  object_name=HIL-2  channels=[7]  sample_time=qc_get_step_size  active=on  vector_output=off  data_type_mode=Inherit via back propagation  data_type=double
  HIL Write Analog : quarc_library/Data Acquisition/Generic/Immediate I//O/HIL Write Analog  object_name=HIL-1  channels=[7]  sample_time=-1  active=off  vector_input=off
  HIL Write Digital : quarc_library/Data Acquisition/Generic/Immediate I//O/HIL Write Digital  object_name=HIL-1  channels=[28:31]  sample_time=-1  active=off  vector_input=off
  Logical Operator : Logic  Operator=NOT  AllPortsSameDT=off  OutDataTypeStr=boolean
  Logical Operator1 : Logic  Operator=OR  AllPortsSameDT=off  OutDataTypeStr=boolean
  Logical Operator2 : Logic  Operator=OR  AllPortsSameDT=off  OutDataTypeStr=boolean
  tics to rad : Gain  Gain=pi/28/2024
  theta_enc : Outport
  theta : Outport  Port=2
  wires:
  4v limit/1 -> HIL Write Analog/1, Display2/1
  Compare To Zero/1 -> Logical Operator/1, Logical Operator1/1
  Abs/1 -> 4v limit/1
  torque/1 -> Compare To Zero/1, Abs/1
  Logical Operator1/1 -> HIL Write Digital/1
  Logical Operator2/1 -> HIL Write Digital/2
  HIL Read Encoder/1 -> tics to rad/1
  HIL Read Analog1/1 -> Display6/1, 1-D Lookup Table3/1
  tics to rad/1 -> theta_enc/1
  enable/1 -> Logical Operator1/2, Logical Operator2/1
  Logical Operator/1 -> Logical Operator2/2
  1-D Lookup Table3/1 -> theta/1

== system MIEM_Adaptive/Right Arm/M14 ==
  torque : Inport
  enable : Inport  Port=2
  1-D Lookup Table3 : Lookup_n-D  NumberOfTableDimensions=1  BreakpointsForDimension1=[1.83 2.47 3.11 3.43 4.14 ]  Table=[-pi/2 -pi/4 0 pi/4 pi/2]  RndMeth=Simplest  InputSameDT=on
  4v limit : Saturate  UpperLimit=4  LowerLimit=0
  Abs : Abs
  Compare To Zero : simulink/Logic and Bit Operations/Compare To Zero  relop=>=  OutDataTypeStr=boolean
  Display : Display
  HIL Read Analog1 : quarc_library/Data Acquisition/Generic/Immediate I//O/HIL Read Analog  object_name=HIL-1  channels=[3]  sample_time=qc_get_step_size  active=on  vector_output=off
  HIL Read Encoder : quarc_library/Data Acquisition/Generic/Immediate I//O/HIL Read Encoder  object_name=HIL-2  channels=[3]  sample_time=qc_get_step_size  active=on  vector_output=off  data_type_mode=Inherit via back propagation  data_type=double
  HIL Write Analog : quarc_library/Data Acquisition/Generic/Immediate I//O/HIL Write Analog  object_name=HIL-1  channels=[3]  sample_time=-1  active=off  vector_input=off
  HIL Write Digital : quarc_library/Data Acquisition/Generic/Immediate I//O/HIL Write Digital  object_name=HIL-1  channels=[12:15]  sample_time=-1  active=off  vector_input=off
  Logical Operator : Logic  Operator=NOT  AllPortsSameDT=off  OutDataTypeStr=boolean
  Logical Operator1 : Logic  Operator=OR  AllPortsSameDT=off  OutDataTypeStr=boolean
  Logical Operator2 : Logic  Operator=OR  AllPortsSameDT=off  OutDataTypeStr=boolean
  tics to rad : Gain  Gain=pi/28/2024
  direction : Outport
  theta : Outport  Port=2
  theta_enc : Outport  Port=3
  wires:
  4v limit/1 -> HIL Write Analog/1
  Compare To Zero/1 -> direction/1, Logical Operator/1, Logical Operator1/1
  Abs/1 -> 4v limit/1
  torque/1 -> Abs/1, Compare To Zero/1
  HIL Read Analog1/1 -> 1-D Lookup Table3/1
  HIL Read Encoder/1 -> tics to rad/1
  Logical Operator/1 -> Logical Operator2/2
  Logical Operator1/1 -> HIL Write Digital/1
  enable/1 -> Logical Operator1/2, Logical Operator2/1
  Logical Operator2/1 -> HIL Write Digital/2
  tics to rad/1 -> theta_enc/1
  1-D Lookup Table3/1 -> theta/1, Display/1

== system MIEM_Adaptive/Right Arm/contoller 22 ==
  qd : Inport
  q : Inport  Port=2
  en : Inport  Port=3
  Constant : Constant  Value=20
  Constant1 : Constant  Value=5e9
  Derivative3 : Derivative
  Derivative4 : Derivative
  Derivative5 : Derivative
  Memory3 : Memory  X0="[-0.0039    0.0394    0.0222   -0.2171]'"
  slotine's adaptive : MATLAB Function  TreatAsAtomicUnit=on
  tau : Outport
  ahat : Outport  Port=2
  wires:
  Derivative4/1 -> slotine's adaptive/6(qddotdot)
  Derivative5/1 -> slotine's adaptive/8(qdot)
  Derivative3/1 -> Derivative4/1, slotine's adaptive/5(qddot)
  slotine's adaptive/2(ahat) -> Memory3/1, ahat/1
  Memory3/1 -> slotine's adaptive/9(ahat_)
  Constant/1 -> slotine's adaptive/2(lambda)
  Constant1/1 -> slotine's adaptive/3(gamma)
  qd/1 -> slotine's adaptive/4(qd), Derivative3/1
  q/1 -> slotine's adaptive/7(q), Derivative5/1
  slotine's adaptive/1(tau) -> tau/1
  en/1 -> slotine's adaptive/1(en)

== system MIEM_Adaptive/Right Arm/controller 21 ==
  qd : Inport
  q : Inport  Port=2
  en : Inport  Port=3
  Constant : Constant  Value=60
  Constant1 : Constant  Value=1e8
  Derivative3 : Derivative
  Derivative4 : Derivative
  Derivative5 : Derivative
  Memory3 : Memory  X0="[3.3914    0.1816    0.3172    0.1486   -5.6249]'"
  slotine's adaptive : MATLAB Function  TreatAsAtomicUnit=on
  tau : Outport
  ahat : Outport  Port=2
  wires:
  Derivative4/1 -> slotine's adaptive/6(qddotdot)
  Derivative5/1 -> slotine's adaptive/8(qdot)
  Derivative3/1 -> Derivative4/1, slotine's adaptive/5(qddot)
  slotine's adaptive/2(ahat) -> Memory3/1, ahat/1
  Memory3/1 -> slotine's adaptive/9(ahat_)
  Constant/1 -> slotine's adaptive/2(lambda)
  Constant1/1 -> slotine's adaptive/3(gamma)
  qd/1 -> slotine's adaptive/4(qd), Derivative3/1
  q/1 -> slotine's adaptive/7(q), Derivative5/1
  slotine's adaptive/1(tau) -> tau/1
  en/1 -> slotine's adaptive/1(en)

== system MIEM_Adaptive/Right Arm/controller 23 ==
  qd : Inport
  q : Inport  Port=2
  en : Inport  Port=3
  Constant : Constant  Value=50
  Constant1 : Constant  Value=1e6
  Derivative3 : Derivative
  Derivative4 : Derivative
  Derivative5 : Derivative
  Memory3 : Memory  X0="[3.3916    0.1811    0.0907   -5.6122]'"
  slotine's adaptive : MATLAB Function  TreatAsAtomicUnit=on
  tau : Outport
  ahat : Outport  Port=2
  wires:
  Derivative4/1 -> slotine's adaptive/6(qddotdot)
  Derivative5/1 -> slotine's adaptive/8(qdot)
  Derivative3/1 -> Derivative4/1, slotine's adaptive/5(qddot)
  slotine's adaptive/2(ahat) -> Memory3/1, ahat/1
  Memory3/1 -> slotine's adaptive/9(ahat_)
  Constant/1 -> slotine's adaptive/2(lambda)
  Constant1/1 -> slotine's adaptive/3(gamma)
  qd/1 -> slotine's adaptive/4(qd), Derivative3/1
  q/1 -> slotine's adaptive/7(q), Derivative5/1
  slotine's adaptive/1(tau) -> tau/1
  en/1 -> slotine's adaptive/1(en)

== system MIEM_Adaptive/Right Arm/controller 24 ==
  qd : Inport
  q : Inport  Port=2
  en : Inport  Port=3
  Constant : Constant  Value=50
  Constant1 : Constant  Value=1e6
  Derivative3 : Derivative
  Derivative4 : Derivative
  Derivative5 : Derivative
  Memory3 : Memory  X0="[0.0008    0.0273    0.0390   -0.0832]'"
  slotine's adaptive : MATLAB Function  TreatAsAtomicUnit=on
  tau : Outport
  ahat : Outport  Port=2
  wires:
  Derivative4/1 -> slotine's adaptive/6(qddotdot)
  Derivative5/1 -> slotine's adaptive/8(qdot)
  Derivative3/1 -> Derivative4/1, slotine's adaptive/5(qddot)
  slotine's adaptive/2(ahat) -> Memory3/1, ahat/1
  Memory3/1 -> slotine's adaptive/9(ahat_)
  Constant/1 -> slotine's adaptive/2(lambda)
  Constant1/1 -> slotine's adaptive/3(gamma)
  qd/1 -> slotine's adaptive/4(qd), Derivative3/1
  q/1 -> slotine's adaptive/7(q), Derivative5/1
  slotine's adaptive/1(tau) -> tau/1
  en/1 -> slotine's adaptive/1(en)

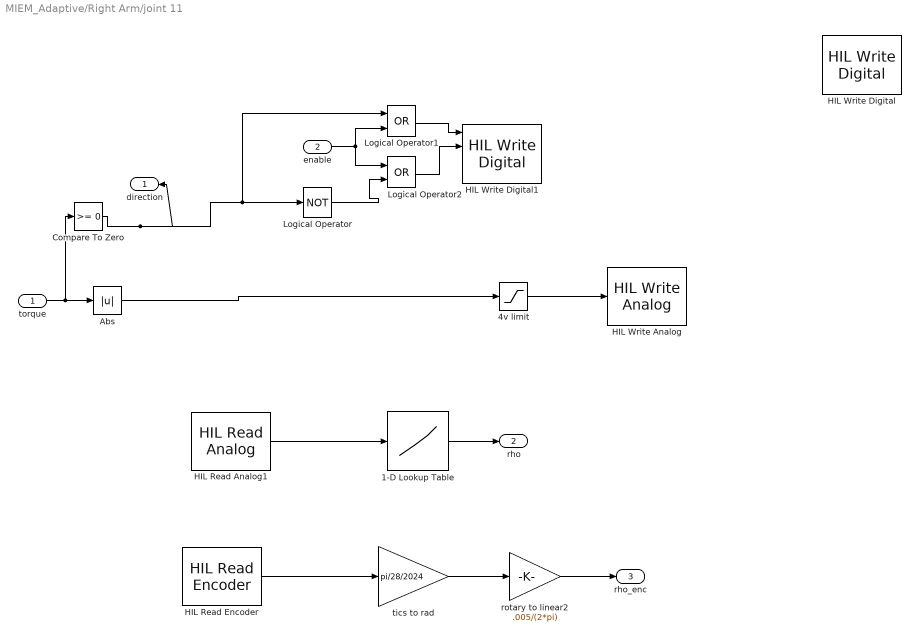
== system MIEM_Adaptive/Right Arm/joint 11 ==
  torque : Inport
  enable : Inport  Port=2
  1-D Lookup Table : Lookup_n-D  NumberOfTableDimensions=1  BreakpointsForDimension1="[.147 .227 .277 .376 .459 .597  .742  .929  1.132  1.36 1.55   1.78  2.078 2.43 2.768  3.016   3.233  3.49  3.78  4.03 4.28]"  Table="[.04 .0375 .0357 .033 .031 .0286 .026  .022  .018  .015  .013  .01  .0088  .0077  .006   .005  .004  .003  .002  .001 0]"  RndMeth=Simplest  InputSameDT=on
  4v limit : Saturate  UpperLimit=4  LowerLimit=0
  Abs : Abs
  Compare To Zero : simulink/Logic and Bit Operations/Compare To Zero  relop=>=  OutDataTypeStr=boolean
  HIL Read Analog1 : quarc_library/Data Acquisition/Generic/Immediate I//O/HIL Read Analog  object_name=HIL-2  channels=[4]  sample_time=qc_get_step_size  active=on  vector_output=off
  HIL Read Encoder : quarc_library/Data Acquisition/Generic/Immediate I//O/HIL Read Encoder  object_name=HIL-2  channels=[0]  sample_time=qc_get_step_size  active=on  vector_output=off  data_type_mode=Inherit via back propagation  data_type=double
  HIL Write Analog : quarc_library/Data Acquisition/Generic/Immediate I//O/HIL Write Analog  object_name=HIL-1  channels=[0]  sample_time=-1  active=off  vector_input=off
  HIL Write Digital : quarc_library/Data Acquisition/Generic/Immediate I//O/HIL Write Digital  object_name=HIL-1  channels=[0:3]  sample_time=-1  active=off  vector_input=off
  HIL Write Digital1 : quarc_library/Data Acquisition/Generic/Immediate I//O/HIL Write Digital  object_name=HIL-1  channels=[40:43]  sample_time=-1  active=off  vector_input=off
  Logical Operator : Logic  Operator=NOT  AllPortsSameDT=off  OutDataTypeStr=boolean
  Logical Operator1 : Logic  Operator=OR  AllPortsSameDT=off  OutDataTypeStr=boolean
  Logical Operator2 : Logic  Operator=OR  AllPortsSameDT=off  OutDataTypeStr=boolean
  rotary to linear2 : Gain  Gain=.005/(2*pi)
  tics to rad : Gain  Gain=pi/28/2024
  direction : Outport
  rho : Outport  Port=2
  rho_enc : Outport  Port=3
  wires:
  4v limit/1 -> HIL Write Analog/1
  Compare To Zero/1 -> direction/1, Logical Operator/1, Logical Operator1/1
  Abs/1 -> 4v limit/1
  torque/1 -> Abs/1, Compare To Zero/1
  HIL Read Analog1/1 -> 1-D Lookup Table/1
  HIL Read Encoder/1 -> tics to rad/1
  Logical Operator/1 -> Logical Operator2/2
  enable/1 -> Logical Operator1/2, Logical Operator2/1
  Logical Operator1/1 -> HIL Write Digital1/1
  Logical Operator2/1 -> HIL Write Digital1/2
  1-D Lookup Table/1 -> rho/1
  tics to rad/1 -> rotary to linear2/1
  rotary to linear2/1 -> rho_enc/1
